simulink model "Pmus_Flow_Younes"  (Simulink 6.4)
settings: Solver=ode45  StartTime=0.0  StopTime=10.0  RelTol=1e-3
values from neighbouring files (symbols this model uses):
  E_CW = 5    [Pleural_Schuessler_IC.m]    (also in Pmus_Flow_Younes_IC.m; Resp_Mech_IC.m; Respiratory_IC.m)
  E_L = 5    [Pleural_Schuessler_IC.m]    (also in Pmus_Flow_Younes_IC.m; Resp_Mech_IC.m; Respiratory_IC.m)
  FlowIC = 0    [Pmus_Flow_Younes_IC.m]    (also in Resp_Mech_IC.m; Respiratory_IC.m)
  G_RespMus = 20    [Pmus_Flow_Younes_IC.m]    (also in Respiratory_IC.m)
  Pt_frcIC1 = 0    [Pmus_Flow_Younes_IC.m]    (also in Resp_Mech_IC.m; Respiratory_IC.m)
  Pt_frcIC2 = 0    [Pmus_Flow_Younes_IC.m]    (also in Resp_Mech_IC.m; Respiratory_IC.m)
  R_AW = 1.27    [Pleural_Schuessler_IC.m]    (also in Pmus_Flow_Younes_IC.m; Resp_Mech_IC.m; Respiratory_IC.m)
  R_CW = 1.03    [Pleural_Schuessler_IC.m]    (also in Pmus_Flow_Younes_IC.m; Resp_Mech_IC.m; Respiratory_IC.m)
  R_L = 1.69    [Pleural_Schuessler_IC.m]    (also in Pmus_Flow_Younes_IC.m; Resp_Mech_IC.m; Respiratory_IC.m)
  RC = 0.06    [Pleural_Schuessler_IC.m]    (also in Pmus_Flow_Younes_IC.m; Resp_Mech_IC.m; Respiratory_IC.m)
  step_size = 0.1    [Pmus_Flow_Younes_IC.m]
  VC = 5    [Pmus_Flow_Younes_IC.m]    (also in Resp_Mech_IC.m; Respiratory_IC.m)
  VtIC = 0    [Pmus_Flow_Younes_IC.m]    (also in Resp_Mech_IC.m; Respiratory_IC.m)
settings Model: LastModifiedBy=CLM
settings OptimizationCC: BlockReduction=off  BooleanDataType=off
settings DebuggingCC: SolverPrmCheckMsg=none  StrictBusMsg=None
settings HardwareCC: TargetUnknown=on

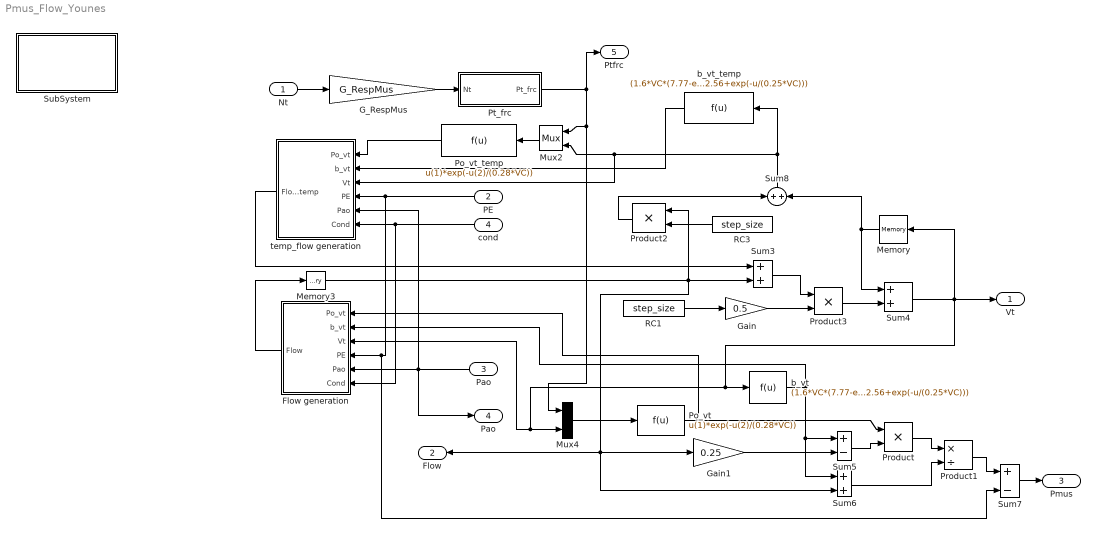
== system Pmus_Flow_Younes ==
  Nt : Inport
  PE : Inport  Orientation=left  Port=2
  Pao : Inport  Orientation=left  Port=3
  "cond " : Inport  Orientation=left  Port=4
  Flow generation : Subsystem  Orientation=left
  G_RespMus : Gain  Gain=G_RespMus  SaturateOnIntegerOverflow=on
  Gain : Gain  Gain=0.5  SaturateOnIntegerOverflow=on
  Gain1 : Gain  Gain=0.25  SaturateOnIntegerOverflow=on
  Memory : Memory  Orientation=left  X0=VtIC  InheritSampleTime=on
  Memory3 : Memory  X0=FlowIC  InheritSampleTime=on
  Mux2 : Mux  Orientation=left  Inputs=2
  Mux4 : Mux  Inputs=2
  Po_vt : Fcn  Expr=u(1)*exp(-u(2)/(0.28*VC))
  Po_vt_temp : Fcn  Orientation=left  Expr=u(1)*exp(-u(2)/(0.28*VC))
  Product : Product  Inputs=**  SaturateOnIntegerOverflow=on  RndMeth=Zero  InputSameDT=on
  Product1 : Product  Inputs=*/  SaturateOnIntegerOverflow=on  RndMeth=Zero  InputSameDT=on
  Product2 : Product  Orientation=left  SaturateOnIntegerOverflow=on  RndMeth=Zero  InputSameDT=on
  Product3 : Product  SaturateOnIntegerOverflow=on  RndMeth=Zero  InputSameDT=on
  Pt_frc : Subsystem
  RC1 : Constant  Value=step_size  OutDataType=sfix(16)  ConRadixGroup=Use specified scaling  OutScaling=2^0  SampleTime=inf  FramePeriod=inf
  RC3 : Constant  Orientation=left  Value=step_size  OutDataType=sfix(16)  ConRadixGroup=Use specified scaling  OutScaling=2^0  SampleTime=inf  FramePeriod=inf
  SubSystem : Subsystem
      settings: OpenFcn=Pmus_Flow_Younes_IC
      mask Display: disp('"double click here"\n to load \nPmus_Flow_Younes \ninitial values');
  Sum3 : Sum  SaturateOnIntegerOverflow=on  InputSameDT=on
  Sum4 : Sum  SaturateOnIntegerOverflow=on  InputSameDT=on
  Sum5 : Sum  Inputs=+-  SaturateOnIntegerOverflow=on  InputSameDT=on
  Sum6 : Sum  SaturateOnIntegerOverflow=on  InputSameDT=on
  Sum7 : Sum  Inputs=+-  SaturateOnIntegerOverflow=on  InputSameDT=on
  Sum8 : Sum  Orientation=up  SaturateOnIntegerOverflow=on  InputSameDT=on
  b_vt : Fcn  Expr=(1.6*VC*(7.77-exp(-u/(0.25*VC))))/(2.56+exp(-u/(0.25*VC)))
  b_vt_temp : Fcn  Orientation=left  Expr=(1.6*VC*(7.77-exp(-u/(0.25*VC))))/(2.56+exp(-u/(0.25*VC)))
  temp_flow generation : Subsystem  Orientation=left
  "Vt " : Outport
  "Flow " : Outport  Orientation=left  Port=2
  Pmus : Outport  Port=3
  "Pao " : Outport  Port=4
  Ptfrc : Outport  Port=5
  wires:
  "cond "/1 -> temp_flow generation/6("Cond "), Flow generation/6("Cond ")
  G_RespMus/1 -> Pt_frc/1(Nt)
  Product3/1 -> Sum4/2
  Sum3/1 -> Product3/1
  Mux2/1 -> Po_vt_temp/1
  Po_vt_temp/1 -> temp_flow generation/1("Po_vt ")
  Gain1/1 -> Sum5/2
  Sum5/1 -> Product/2
  Product/1 -> Product1/1
  Sum6/1 -> Product1/2
  Mux4/1 -> Po_vt/1
  b_vt_temp/1 -> temp_flow generation/2(b_vt)
  temp_flow generation/1(Flow_temp) -> Sum3/1
  Memory3/1 -> Product2/1, Sum3/2, "Flow "/1, Sum6/2, Gain1/1
  Sum4/1 -> b_vt/1, Flow generation/3(Vt), Mux4/2, Memory/1, "Vt "/1
  PE/1 -> Sum7/2, Flow generation/4(PE), temp_flow generation/4(PE)
  Pt_frc/1(Pt_frc) -> Mux2/1, Mux4/1, Ptfrc/1
  b_vt/1 -> Flow generation/2(b_vt), Sum6/1, Sum5/1
  Po_vt/1 -> Flow generation/1("Po_vt "), Product/1
  Product1/1 -> Sum7/1
  Memory/1 -> Sum8/2, Sum4/1
  Flow generation/1(Flow) -> Memory3/1
  Sum8/1 -> b_vt_temp/1, temp_flow generation/3(Vt), Mux2/2
  RC3/1 -> Product2/2
  Gain/1 -> Product3/2
  Sum7/1 -> Pmus/1
  Nt/1 -> G_RespMus/1
  Product2/1 -> Sum8/1
  RC1/1 -> Gain/1
  Pao/1 -> temp_flow generation/5("Pao "), "Pao "/1, Flow generation/5("Pao ")

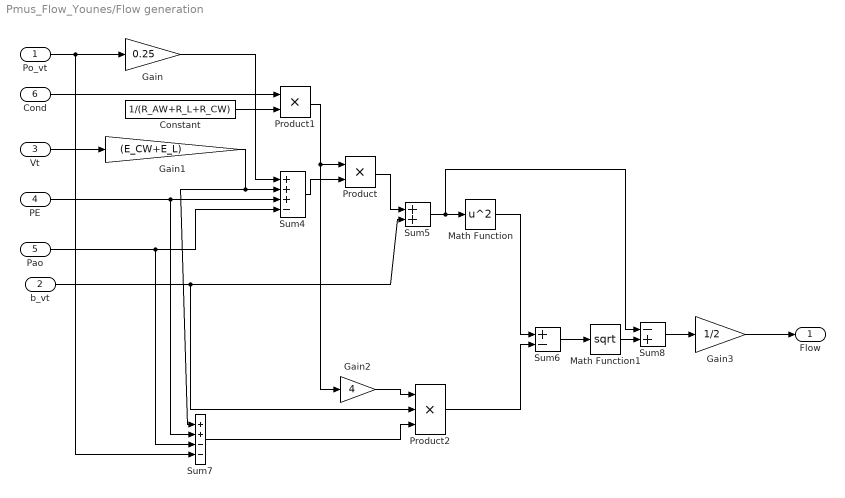
== system Pmus_Flow_Younes/Flow generation ==
  "Po_vt " : Inport
  b_vt : Inport  Port=2
  Vt : Inport  Port=3
  PE : Inport  Port=4
  "Pao " : Inport  Port=5
  "Cond " : Inport  Port=6
  Constant : Constant  Value=1/(R_AW+R_L+R_CW)  OutDataType=sfix(16)  ConRadixGroup=Use specified scaling  OutScaling=2^0  SampleTime=inf  FramePeriod=inf
  Gain : Gain  Gain=0.25  SaturateOnIntegerOverflow=on
  Gain1 : Gain  Gain=(E_CW+E_L)  SaturateOnIntegerOverflow=on
  Gain2 : Gain  Gain=4  SaturateOnIntegerOverflow=on
  Gain3 : Gain  Gain=1/2  SaturateOnIntegerOverflow=on
  Math Function : Math  Operator=square  SaturateOnIntegerOverflow=on
  Math Function1 : Math  Operator=sqrt  SaturateOnIntegerOverflow=on
  Product : Product  SaturateOnIntegerOverflow=on  RndMeth=Zero  InputSameDT=on
  Product1 : Product  SaturateOnIntegerOverflow=on  RndMeth=Zero  InputSameDT=on
  Product2 : Product  Inputs=3  SaturateOnIntegerOverflow=on  RndMeth=Zero  InputSameDT=on
  Sum4 : Sum  Inputs=+++-  SaturateOnIntegerOverflow=on  InputSameDT=on
  Sum5 : Sum  SaturateOnIntegerOverflow=on  InputSameDT=on
  Sum6 : Sum  Inputs=+-  SaturateOnIntegerOverflow=on  InputSameDT=on
  Sum7 : Sum  Inputs=++--  SaturateOnIntegerOverflow=on  InputSameDT=on
  Sum8 : Sum  Inputs=-+  SaturateOnIntegerOverflow=on  InputSameDT=on
  Flow : Outport
  wires:
  Constant/1 -> Product1/2
  "Cond "/1 -> Product1/1
  Product1/1 -> Gain2/1, Product/1
  Vt/1 -> Gain1/1
  Gain/1 -> Sum4/1
  Sum4/1 -> Product/2
  Product/1 -> Sum5/1
  Math Function/1 -> Sum6/1
  Gain2/1 -> Product2/1
  b_vt/1 -> Sum5/2, Product2/2
  Sum7/1 -> Product2/3
  Gain1/1 -> Sum4/2, Sum7/1
  PE/1 -> Sum4/3, Sum7/2
  "Pao "/1 -> Sum4/4, Sum7/3
  "Po_vt "/1 -> Gain/1, Sum7/4
  Product2/1 -> Sum6/2
  Sum6/1 -> Math Function1/1
  Math Function1/1 -> Sum8/2
  Sum5/1 -> Math Function/1, Sum8/1
  Sum8/1 -> Gain3/1
  Gain3/1 -> Flow/1

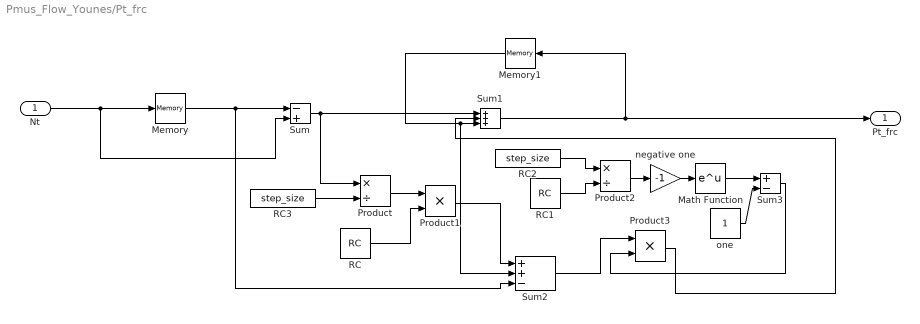
== system Pmus_Flow_Younes/Pt_frc ==
  Nt : Inport
  Math Function : Math  SaturateOnIntegerOverflow=on
  Memory : Memory  X0=Pt_frcIC1  InheritSampleTime=on
  Memory1 : Memory  Orientation=left  X0=Pt_frcIC2  InheritSampleTime=on
  Product : Product  Inputs=*/  SaturateOnIntegerOverflow=on  RndMeth=Zero  InputSameDT=on
  Product1 : Product  Inputs=**  SaturateOnIntegerOverflow=on  RndMeth=Zero  InputSameDT=on
  Product2 : Product  Inputs=*/  SaturateOnIntegerOverflow=on  RndMeth=Zero  InputSameDT=on
  Product3 : Product  Inputs=**  SaturateOnIntegerOverflow=on  RndMeth=Zero  InputSameDT=on
  RC : Constant  Value=RC  OutDataType=sfix(16)  ConRadixGroup=Use specified scaling  OutScaling=2^0  SampleTime=inf  FramePeriod=inf
  RC1 : Constant  Value=RC  OutDataType=sfix(16)  ConRadixGroup=Use specified scaling  OutScaling=2^0  SampleTime=inf  FramePeriod=inf
  RC2 : Constant  Value=step_size  OutDataType=sfix(16)  ConRadixGroup=Use specified scaling  OutScaling=2^0  SampleTime=inf  FramePeriod=inf
  RC3 : Constant  Value=step_size  OutDataType=sfix(16)  ConRadixGroup=Use specified scaling  OutScaling=2^0  SampleTime=inf  FramePeriod=inf
  Sum : Sum  Inputs=-+  SaturateOnIntegerOverflow=on  InputSameDT=on
  Sum1 : Sum  Inputs=+++  SaturateOnIntegerOverflow=on  InputSameDT=on
  Sum2 : Sum  Inputs=++-  SaturateOnIntegerOverflow=on  InputSameDT=on
  Sum3 : Sum  Inputs=+-  SaturateOnIntegerOverflow=on  InputSameDT=on
  negative one : Gain  Gain=-1  SaturateOnIntegerOverflow=on
  one : Constant  Value=1  OutDataType=sfix(16)  ConRadixGroup=Use specified scaling  OutScaling=2^0  SampleTime=inf  FramePeriod=inf
  Pt_frc : Outport
  wires:
  Nt/1 -> Sum/2, Memory/1
  Sum/1 -> Sum1/1, Product/1
  RC3/1 -> Product/2
  Product/1 -> Product1/1
  RC/1 -> Product1/2
  Product1/1 -> Sum2/1
  Memory/1 -> Sum/1, Sum2/3
  RC2/1 -> Product2/1
  RC1/1 -> Product2/2
  Product2/1 -> negative one/1
  negative one/1 -> Math Function/1
  Math Function/1 -> Sum3/1
  one/1 -> Sum3/2
  Sum3/1 -> Product3/2
  Product3/1 -> Sum1/2
  Sum1/1 -> Pt_frc/1, Memory1/1
  Sum2/1 -> Product3/1
  Memory1/1 -> Sum1/3, Sum2/2

== system Pmus_Flow_Younes/SubSystem ==

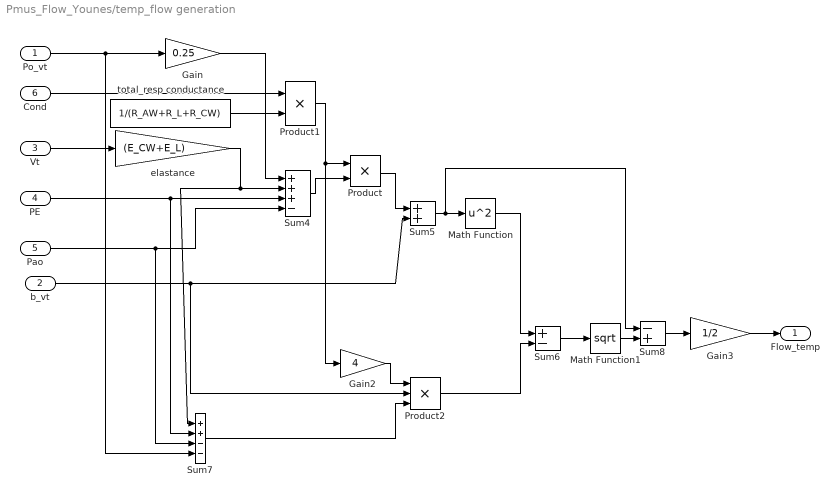
== system Pmus_Flow_Younes/temp_flow generation ==
  "Po_vt " : Inport
  b_vt : Inport  Port=2
  Vt : Inport  Port=3
  PE : Inport  Port=4
  "Pao " : Inport  Port=5
  "Cond " : Inport  Port=6
  Gain : Gain  Gain=0.25  SaturateOnIntegerOverflow=on
  Gain2 : Gain  Gain=4  SaturateOnIntegerOverflow=on
  Gain3 : Gain  Gain=1/2  SaturateOnIntegerOverflow=on
  Math Function : Math  Operator=square  SaturateOnIntegerOverflow=on
  Math Function1 : Math  Operator=sqrt  SaturateOnIntegerOverflow=on
  Product : Product  SaturateOnIntegerOverflow=on  RndMeth=Zero  InputSameDT=on
  Product1 : Product  SaturateOnIntegerOverflow=on  RndMeth=Zero  InputSameDT=on
  Product2 : Product  Inputs=3  SaturateOnIntegerOverflow=on  RndMeth=Zero  InputSameDT=on
  Sum4 : Sum  Inputs=+++-  SaturateOnIntegerOverflow=on  InputSameDT=on
  Sum5 : Sum  SaturateOnIntegerOverflow=on  InputSameDT=on
  Sum6 : Sum  Inputs=+-  SaturateOnIntegerOverflow=on  InputSameDT=on
  Sum7 : Sum  Inputs=++--  SaturateOnIntegerOverflow=on  InputSameDT=on
  Sum8 : Sum  Inputs=-+  SaturateOnIntegerOverflow=on  InputSameDT=on
  elastance : Gain  Gain=(E_CW+E_L)  SaturateOnIntegerOverflow=on
  total_resp conductance : Constant  Value=1/(R_AW+R_L+R_CW)  OutDataType=sfix(16)  ConRadixGroup=Use specified scaling  OutScaling=2^0  SampleTime=inf  FramePeriod=inf
  Flow_temp : Outport
  wires:
  Gain/1 -> Sum4/1
  total_resp conductance/1 -> Product1/2
  "Cond "/1 -> Product1/1
  Product1/1 -> Gain2/1, Product/1
  Gain3/1 -> Flow_temp/1
  Sum8/1 -> Gain3/1
  Sum5/1 -> Sum8/1, Math Function/1
  Math Function1/1 -> Sum8/2
  Sum6/1 -> Math Function1/1
  Product2/1 -> Sum6/2
  "Po_vt "/1 -> Sum7/4, Gain/1
  "Pao "/1 -> Sum7/3, Sum4/4
  PE/1 -> Sum7/2, Sum4/3
  elastance/1 -> Sum7/1, Sum4/2
  Sum7/1 -> Product2/3
  b_vt/1 -> Product2/2, Sum5/2
  Gain2/1 -> Product2/1
  Math Function/1 -> Sum6/1
  Product/1 -> Sum5/1
  Sum4/1 -> Product/2
  Vt/1 -> elastance/1
